simulink model "MBE_Simulation_04_Template_14_11_final"  (R2017b)
settings: Solver=FixedStepAuto  StartTime=0.0  StopTime=inf  FixedStep=0.05  RelTol=1e-3
libraries: simulink x67, canmsglib x4, instrumentlib x2, realtime_pacer_lib x1, hdlsllib x1
(part 4 of 4)

== stateflow chart MBE_Simulation_04_Template_14_11_final/WischerSensorBox/WS_Box_Applikation/WischerSteuerung ==
  state Dummy8 [commented out]
    entry:
    SM_A=true;
    SM_B=false;
    SM_C=false;
    SM_D=false;
    WW_LED=true;
  state Dummy7 [commented out]
    entry:
    SM_A=true;
    SM_B=true;
    SM_C=false;
    SM_D=false;
    WW_LED=true;
  state State_Intervall_Langsam [commented out]
  state State_Wisch_Wasch [commented out]
  state Dummy6 [commented out]
    entry:
    SM_A=true;
    SM_B=false;
    SM_C=false;
    SM_D=true;
    WW_LED=true;
  state Dummy5 [commented out]
    entry:
    SM_A=false;
    SM_B=true;
    SM_C=false;
    SM_D=false;
    WW_LED=true;
  state State_Intervall_Schnell [commented out]
  state State_OFF [commented out]
  state State_Tipp [commented out]
  state Dummy10 [commented out]
    entry:
    SM_A=false;
    SM_B=false;
    SM_C=false;
    SM_D=true;
    WW_LED=true;
  state Dummy11 [commented out]
    entry:
    SM_A=false;
    SM_B=true;
    SM_C=true;
    SM_D=false;
    WW_LED=true;
  state Dummy12 [commented out]
    entry:
    SM_A=false;
    SM_B=false;
    SM_C=true;
    SM_D=true;
    WW_LED=true;
  state Dummy9 [commented out]
    entry:
    SM_A=false;
    SM_B=false;
    SM_C=true;
    SM_D=false;
    WW_LED=true;
  state State_Dauer_Schnell [commented out]
  state State_Dauer_Langsam [commented out]
  state Wischer
    en, du: wisher_cnt = 0
    state Dauer_Schnell
      en, du: wischen = true
      frequency = 0
      wisher_delay = 0
    state Dauer_Langsam
      en, du: wischen = true
      frequency = 0.1
      wisher_delay = 0
    state OFF
      en, du: wischen = false
      wisher_delay = 0
    state Intervall_Langsam
      en, du: wischen = true
      frequency = 0.1
      wisher_delay = 4
    state Intervall_Schnell
      en, du: wischen = true
      frequency = 0.1
      wisher_delay = 2
    state Tipp
      en, du: wischen = true
      frequency = 0
      wisher_delay = 0
    state Wisch_Wasch_Aktivierung
      en, du:
      if SchlossZustand == true
      WischWaschActive = true
      end
      Interrupt = false
      frequency = 0.1
      wisher_delay = 0
      wisher_cnt = 3
    (junction 402) -> Dauer_Schnell [order 3] : [Wischer_Dauer_II]
    (junction 402) -> Dauer_Langsam [order 2] : [Wischer_Dauer_I]
    (junction 402) -> OFF [order 7]
    (default) -> (junction 402)
    Wischer -> (junction 402) [order 1]
    (junction 402) -> Intervall_Langsam [order 5] : [Wischer_Intervall_I]
    (junction 402) -> Intervall_Schnell [order 4] : [Wischer_Intervall_II]
    (junction 402) -> Tipp [order 6] : [Wischer_Tipp]
    (junction 402) -> Wisch_Wasch_Aktivierung [order 1] : [WischWasch || Interrupt]
  state State_MotorWischen1
    en, du: if counter==27
    linkslauf = true
    end
    if WischWasch == true
    Interrupt = true
    end
    state Dummy
      entry:
      SM_A=true;
      SM_B=true;
      SM_C=false;
      SM_D=false;
    state Dummy1
      entry:
      SM_A=false;
      SM_B=true;
      SM_C=true;
      SM_D=false;
    state Dummy3
      entry:
      SM_A=true;
      SM_B=false;
      SM_C=false;
      SM_D=true;
    state Dummy2
      entry:
      SM_A=false;
      SM_B=false;
      SM_C=true;
      SM_D=true;
    (default) -> State_MotorWischen1.Dummy
    State_MotorWischen1.Dummy -> State_MotorWischen1.Dummy1 [order 1] : [linkslauf == 0 && counter <= 27 && after(frequency,sec)]{counter = counter + 1}
    State_MotorWischen1.Dummy1 -> State_MotorWischen1.Dummy [order 2] : [linkslauf == 1 && counter <= 54 && after(frequency,sec)]{counter = counter + 1}
    State_MotorWischen1.Dummy3 -> State_MotorWischen1.Dummy [order 1] : [linkslauf == 0 && counter <= 27 && after(frequency,sec)]{counter = counter + 1}
    State_MotorWischen1.Dummy -> State_MotorWischen1.Dummy3 [order 2] : [linkslauf == 1 && counter <= 54 && after(frequency,sec)]{counter = counter + 1}
    State_MotorWischen1.Dummy2 -> State_MotorWischen1.Dummy1 [order 2] : [linkslauf == 1 && counter <= 54 && after(frequency,sec)]{counter = counter + 1}
    State_MotorWischen1.Dummy1 -> State_MotorWischen1.Dummy2 [order 1] : [linkslauf == 0 && counter <= 27 && after(frequency,sec)]{counter = counter + 1}
    State_MotorWischen1.Dummy3 -> State_MotorWischen1.Dummy2 [order 2] : [linkslauf == 1 && counter <= 54 && after(frequency,sec)]{counter = counter + 1}
    State_MotorWischen1.Dummy2 -> State_MotorWischen1.Dummy3 [order 1] : [linkslauf == 0 && counter <= 27 && after(frequency,sec)]{counter = counter + 1}
  state State_MotorWischen [commented out]
    en, du: WW_LED = true
    if counter==27
    linkslauf = true
    end
    state Dummy [commented out]
      entry:
      SM_A=true;
      SM_B=true;
      SM_C=false;
      SM_D=false;
    state Dummy1 [commented out]
      entry:
      SM_A=false;
      SM_B=true;
      SM_C=true;
      SM_D=false;
    state Dummy3 [commented out]
      entry:
      SM_A=true;
      SM_B=false;
      SM_C=false;
      SM_D=true;
    state Dummy2 [commented out]
      entry:
      SM_A=false;
      SM_B=false;
      SM_C=true;
      SM_D=true;
    (default) -> State_MotorWischen.Dummy [commented out]
    State_MotorWischen.Dummy -> State_MotorWischen.Dummy1 [commented out] : [linkslauf == 0 && counter <= 27 && after(frequency,sec)]{counter = counter + 1}
    State_MotorWischen.Dummy1 -> State_MotorWischen.Dummy [commented out] : [linkslauf == 1 && counter > 0 && after(frequency,sec)]{counter = counter - 1}
    State_MotorWischen.Dummy3 -> State_MotorWischen.Dummy [commented out] : [linkslauf == 0 && counter <= 27 && after(frequency,sec)]{counter = counter + 1}
    State_MotorWischen.Dummy -> State_MotorWischen.Dummy3 [commented out] : [linkslauf == 1 && counter > 0 && after(frequency,sec)]{counter = counter - 1}
    State_MotorWischen.Dummy2 -> State_MotorWischen.Dummy1 [commented out] : [linkslauf == 1 && counter > 0 && after(frequency,sec)]{counter = counter - 1}
    State_MotorWischen.Dummy1 -> State_MotorWischen.Dummy2 [commented out] : [linkslauf == 0 && counter <= 27 && after(frequency,sec)]{counter = counter + 1}
    State_MotorWischen.Dummy3 -> State_MotorWischen.Dummy2 [commented out] : [linkslauf == 1 && counter > 0 && after(frequency,sec)]{counter = counter - 1}
    State_MotorWischen.Dummy2 -> State_MotorWischen.Dummy3 [commented out] : [linkslauf == 0 && counter <= 27 && after(frequency,sec)]{counter = counter + 1}
  state Dummy4 [commented out]
    entry:
    SM_A=true;
    SM_B=false;
    SM_C=true;
    SM_D=false;
    WW_LED=true;
  state State_Delay
  state Wisch_Wasch_LED
    en, du: WW_LED = true
  state Wisch_Wasch
    en, du:
    WW_LED = false
  (default) -> Dummy8 [commented out]
  Dummy6 -> Dummy8 [commented out] : [after(0.5,sec)]
  Dummy8 -> Dummy7 [commented out] : [after(0.5,sec)]
  Dummy7 -> Dummy5 [commented out] : [after(0.5,sec)]
  State_OFF -> State_Wisch_Wasch [commented out]
  State_Wisch_Wasch -> State_OFF [commented out]
  State_OFF -> State_Intervall_Langsam [commented out]
  State_Intervall_Langsam -> State_OFF [commented out]
  Dummy10 -> Dummy6 [commented out] : [after(0.5,sec)]
  (default) -> State_OFF [commented out]
  Dummy5 -> Dummy11 [commented out] : [after(0.5,sec)]
  State_OFF -> State_Intervall_Schnell [commented out]
  State_Intervall_Schnell -> State_OFF [commented out]
  State_Tipp -> State_OFF [commented out]
  State_Dauer_Langsam -> State_OFF [commented out]
  State_OFF -> State_Tipp [commented out] : [Wischer_Tipp == true]
  State_OFF -> State_Dauer_Langsam [commented out]
  State_Dauer_Schnell -> State_OFF [commented out]
  State_OFF -> State_Dauer_Schnell [commented out]
  Dummy12 -> Dummy10 [commented out] : [after(0.5,sec)]
  Dummy11 -> Dummy9 [commented out] : [after(0.5,sec)]
  Dummy9 -> Dummy12 [commented out] : [after(0.5,sec)]
  (default) -> Wischer : {WischWaschActive = false, Interrupt = false}
  (default) -> State_MotorWischen [commented out] : {counter = 0, frequency = 0.1, linkslauf = false}
  Wischer -> State_MotorWischen1 [order 2] : [wischen == true]{counter = 0, linkslauf = false}
  (default) -> Dummy4 [commented out]
  State_MotorWischen1 -> State_Delay : [counter == 55]{wischen = false}
  Wisch_Wasch -> State_MotorWischen1 [order 1] : [wisher_cnt > 0]{counter = 0, linkslauf = false}
  State_Delay -> Wischer [order 2] : after(wisher_delay, sec)
  State_Delay -> Wisch_Wasch [order 1] : [WischWaschActive == true]{wisher_cnt = wisher_cnt - 1}
  Wisch_Wasch -> Wischer [order 2] : [wisher_cnt == 0]{WischWaschActive = false}
  Wischer -> Wisch_Wasch_LED [order 1] : [WischWaschActive == true]
  Wisch_Wasch_LED -> Wisch_Wasch : [after(2,sec)]
  data: Wischer_Tipp input; Wischer_Intervall_I input; Wischer_Intervall_II input; Wischer_Dauer_I input; Wischer_Dauer_II input; WischWasch input; SM_A output; SM_B output; SM_C output; SM_D output; WW_LED output; Steps local; Forward local; StepTime local; StepTime1 local; wisher_delay local double; wisher_cnt local uint8; wisher_dir local boolean; wisher_active local boolean; wisher_timeout local double; frequency local double; counter local double; linkslauf local boolean; Pause local double; wischen local boolean; WischWaschActive local boolean; Interrupt local boolean; SchlossZustand input uint16

== stateflow chart MBE_Simulation_04_Template_14_11_final/WischerSensorBox/WS_Box_Applikation/ScheibenheizungsSteuerung ==
  state State_WaitForDeactivateButton
    entry: SH_LED=false
  state State_OFF
    entry:
    SH_LED=false
  state State_Auto
    entry: SH_LED=true
  state State_Manuell
    entry:
    SH_LED=true
  State_Manuell -> State_WaitForDeactivateButton [order 1] : [after(30,sec)]
  State_WaitForDeactivateButton -> State_OFF : [Scheibenheizung == false]
  (default) -> State_OFF
  State_OFF -> State_Auto [order 2] : [Scheibenheizung_Auto == true && Temperatur < 62]
  State_Manuell -> State_OFF [order 2] : [Scheibenheizung == false]
  State_OFF -> State_Manuell [order 1] : [Scheibenheizung == true]
  State_Auto -> State_OFF : [Scheibenheizung_Auto == false || after(30,sec)]
  data: Scheibenheizung input; Scheibenheizung_Auto input; Temperatur input; SH_LED output

== matlab function MBE_Simulation_04_Template_14_11_final/MLF-VirtualPlatform Setup/Subsystem/Triggered Subsystem/MATLAB Function1 ==
  data: alarmAlarmButton input; alarmAlarmLight input; alarmGenericButton input; alarmGenericLightDown input; alarmGenericLightLeft input; alarmGenericLightRight input; alarmGenericLightUp input; alarmLockButton input; alarmLockLight input; lightBacklight input; lightBrakelight input; lightDaylight input; json_output output size=4096; lightFoglightLeft input; lightFoglightRight input; lightGenericButton input; lightGenericLightDown input; lightGenericLightLeft input; lightGenericLightRight input; lightGenericLightUp input; lightIndicatorLeft input; lightIndicatorRight input; lightLowerBeamHeadlight input; lightReverselight input; lightUpperBeamHeadlight input; windshieldDistanceSensor input; windshieldGenericButton input; windshieldGenericLightDown input; windshieldGenericLightLeft input; windshieldGenericLightRight input; windshieldGenericLightUp input; windshieldHeater input; windshieldLightSensor input; windshieldWasherPump input; windshieldWiperA input; windshieldWiperB input; windshieldWiperC input; windshieldWiperD input
function json_output = fcn( ...
    alarmAlarmButton, ...
    alarmAlarmLight, ...
    alarmGenericButton, ...
    alarmGenericLightDown, ...
    alarmGenericLightLeft, ...
    alarmGenericLightRight, ...
    alarmGenericLightUp, ...
    alarmLockButton, ...
    alarmLockLight, ...
    lightBacklight, ...
    lightBrakelight, ...
    lightDaylight, ...
    lightFoglightLeft, ...
    lightFoglightRight, ...
    lightGenericButton, ...
    lightGenericLightDown, ...
    lightGenericLightLeft, ...
    lightGenericLightRight, ...
    lightGenericLightUp, ...
    lightIndicatorLeft, ...
    lightIndicatorRight, ...
    lightLowerBeamHeadlight, ...
    lightReverselight, ...
    lightUpperBeamHeadlight, ...
    windshieldDistanceSensor, ...
    windshieldGenericButton, ...
    windshieldGenericLightDown, ...
    windshieldGenericLightLeft, ...
    windshieldGenericLightRight, ...
    windshieldGenericLightUp, ...
    windshieldHeater, ...
    windshieldLightSensor, ...
    windshieldWasherPump, ...
    windshieldWiperA, ...
    windshieldWiperB, ...
    windshieldWiperC, ...
    windshieldWiperD)

coder.extrinsic('jsonencode')

% Allocate output array size an initialize with zeroes
json_output = zeros(4096,1,'uint8');


% Prepare the data
json_struct = struct(...
    'alarmAlarmButton', alarmAlarmButton, ...
    'alarmAlarmLight', alarmAlarmLight, ...
    'alarmGenericButton', alarmGenericButton, ...
    'alarmGenericLightDown', alarmGenericLightDown, ...
    'alarmGenericLightLeft', alarmGenericLightLeft, ...
    'alarmGenericLightRight', alarmGenericLightRight, ...
    'alarmGenericLightUp', alarmGenericLightUp, ...
    'alarmLockButton', alarmLockButton, ...
    'alarmLockLight', alarmLockLight, ...
    'lightBacklight',lightBacklight, ...
    'lightBrakelight',lightBrakelight, ...
    'lightDaylight',lightDaylight, ...
    'lightFoglightLeft', lightFoglightLeft, ...
    'lightFoglightRight', lightFoglightRight, ...
    'lightGenericButton', lightGenericButton, ...
    'lightGenericLightDown', lightGenericLightDown, ...
    'lightGenericLightLeft', lightGenericLightLeft, ...
    'lightGenericLightRight', lightGenericLightRight, ...
    'lightGenericLightUp', lightGenericLightUp, ...
    'lightIndicatorLeft', lightIndicatorLeft, ...
    'lightIndicatorRight', lightIndicatorRight, ...
    'lightLowerBeamHeadlight', lightLowerBeamHeadlight, ...
    'lightReverselight', lightReverselight, ...
    'lightUpperBeamHeadlight', lightUpperBeamHeadlight, ...
    'windshieldDistanceSensor', windshieldDistanceSensor, ...
    'windshieldGenericButton', windshieldGenericButton, ...
    'windshieldGenericLightDown', windshieldGenericLightDown, ...
    'windshieldGenericLightLeft', windshieldGenericLightLeft, ...
    'windshieldGenericLightRight', windshieldGenericLightRight, ...
    'windshieldGenericLightUp', windshieldGenericLightUp, ...
    'windshieldHeater', windshieldHeater, ...
    'windshieldLightSensor', windshieldLightSensor, ...
    'windshieldWasherPump', windshieldWasherPump, ...
    'windshieldWiperA', windshieldWiperA, ...
    'windshieldWiperB', windshieldWiperB, ...
    'windshieldWiperC', windshieldWiperC, ...
    'windshieldWiperD', windshieldWiperD ...
)

% Create json string from data
json_string = jsonencode(json_struct)

% Get length of final json string
len = uint16(0)
len = uint16(length(json_string))

% Copy json string char by char to output string
for i = 1:len
    json_output(i) = uint8(json_string(i));
end

json_output(len+1) = uint8(10)

== stateflow chart MBE_Simulation_04_Template_14_11_final/LeuchtenBlinkerBox/LB_Box_Applikation/Steuerung_Licht1 ==
  state on
    state up
      entry:
      up=true;
      left=false;
      right=false;
      down=false;
    state left
      entry:
      up=false;
      left=true;
      right=false;
      down=false;
    state right
      entry:
      up=false;
      left=false;
      right=true;
      down=false;
    state down
      entry:
      up=false;
      left=false;
      right=false;
      down=true;
    (default) -> up
    left -> up : [after(0.5,sec)]
    up -> right : [after(0.5,sec)]
    down -> left : [after(0.5,sec)]
    right -> down : [after(0.5,sec)]
  state off
    entry:
    up=false;
    left=false;
    right=false;
    down=false;
  (default) -> off
  off -> on : [button]
  on -> off : [~button]
  data: down output boolean; left output boolean; right output boolean; up output boolean; button input boolean

== stateflow chart MBE_Simulation_04_Template_14_11_final/SchlossAlarmBox/SA_Box_Applikation/Generic_Lights_Example ==
  state on
    state up
      entry:
      up=true;
      left=false;
      right=false;
      down=false;
    state left
      entry:
      up=false;
      left=true;
      right=false;
      down=false;
    state right
      entry:
      up=false;
      left=false;
      right=true;
      down=false;
    state down
      entry:
      up=false;
      left=false;
      right=false;
      down=true;
    (default) -> up
    left -> up : [after(0.5,sec)]
    up -> right : [after(0.5,sec)]
    down -> left : [after(0.5,sec)]
    right -> down : [after(0.5,sec)]
  state off
    entry:
    up=false;
    left=false;
    right=false;
    down=false;
  (default) -> off
  off -> on : [button]
  on -> off : [~button]
  data: down output boolean; left output boolean; right output boolean; up output boolean; button input boolean

== stateflow chart MBE_Simulation_04_Template_14_11_final/LeuchtenBlinkerBox/LB_Box_Applikation/Generic_Lights_Example ==
  state on
    state up
      entry:
      up=true
      left=false
      right=false
      down=false
    state left
      entry:
      up=false
      left=true
      right=false
      down=false
    state right
      entry:
      up=false
      left=false
      right=true
      down=false
    state down
      entry:
      up=false
      left=false
      right=false
      down=true
    (default) -> up
    left -> up : [after(0.5,sec)]
    up -> right : [after(0.5,sec)]
    down -> left : [after(0.5,sec)]
    right -> down : [after(0.5,sec)]
  state off
    entry:
    up=false
    left=false
    right=false
    down=false
  (default) -> off
  off -> on : [button]
  on -> off : [~button]
  data: down output boolean; left output boolean; right output boolean; up output boolean; button input boolean

== stateflow chart MBE_Simulation_04_Template_14_11_final/WischerSensorBox/WS_Box_Applikation/Generic_Lights_Example ==
  state on
    state up
      entry:
      up=true;
      left=false;
      right=false;
      down=false;
    state left
      entry:
      up=false;
      left=true;
      right=false;
      down=false;
    state right
      entry:
      up=false;
      left=false;
      right=true;
      down=false;
    state down
      entry:
      up=false;
      left=false;
      right=false;
      down=true;
    (default) -> up
    left -> up : [after(0.5,sec)]
    up -> right : [after(0.5,sec)]
    down -> left : [after(0.5,sec)]
    right -> down : [after(0.5,sec)]
  state off
    entry:
    up=false;
    left=false;
    right=false;
    down=false;
  (default) -> off
  off -> on : [button]
  on -> off : [~button]
  data: down output boolean; left output boolean; right output boolean; up output boolean; button input boolean

== matlab function MBE_Simulation_04_Template_14_11_final/MLF-VirtualPlatform Setup/Subsystem2/Triggered Subsystem/MATLAB Function ==
  data: json_input input; alarmAlarmButton output; alarmAlarmLight output; alarmGenericButton output; alarmGenericLightDown output; alarmGenericLightLeft output; alarmGenericLightRight output; alarmGenericLightUp output; alarmLockButton output; alarmLockLight output; cockpitAlarmReset output; cockpitBrake output; cockpitIgnition output; cockpitIndicator output; cockpitLightSwitch output; cockpitSteeringAngleDeg output; cockpitTemperature output; cockpitVelocity output; cockpitWarnLight output; cockpitWindshieldHeater output; cockpitWindshieldWasherMode output; cockpitWindshieldWasherPump output; lightBacklight output; lightBrakelight output; lightDaylight output; lightFoglightLeft output; lightFoglightRight output; lightGenericButton output; lightGenericLightDown output; lightGenericLightLeft output; lightGenericLightRight output; lightGenericLightUp output; lightIndicatorLeft output; lightIndicatorRight output; lightLowerBeamHeadlight output; lightReverselight output; lightUpperBeamHeadlight output; windshieldDistanceSensor output; windshieldGenericButton output; windshieldGenericLightDown output; windshieldGenericLightLeft output; windshieldGenericLightRight output; windshieldGenericLightUp output; windshieldHeater output; windshieldLightSensor output; windshieldWasherPump output; windshieldWiperA output; windshieldWiperB output; windshieldWiperC output; windshieldWiperD output
function [ ...
    alarmAlarmButton, ...
    alarmAlarmLight, ...
    alarmGenericButton, ...
    alarmGenericLightDown, ...
    alarmGenericLightLeft, ...
    alarmGenericLightRight, ...
    alarmGenericLightUp, ...
    alarmLockButton, ...
    alarmLockLight, ...
    cockpitAlarmReset, ...
    cockpitBrake, ...
    cockpitIgnition, ...
    cockpitIndicator, ...
    cockpitLightSwitch, ...
    cockpitSteeringAngleDeg, ...
    cockpitTemperature, ...
    cockpitVelocity, ...
    cockpitWarnLight, ...
    cockpitWindshieldHeater, ...
    cockpitWindshieldWasherMode, ...
    cockpitWindshieldWasherPump, ...
    lightBacklight, ...
    lightBrakelight, ...
    lightDaylight, ...
    lightFoglightLeft, ...
    lightFoglightRight, ...
    lightGenericButton, ...
    lightGenericLightDown, ...
    lightGenericLightLeft, ...
    lightGenericLightRight, ...
    lightGenericLightUp, ...
    lightIndicatorLeft, ...
    lightIndicatorRight, ...
    lightLowerBeamHeadlight, ...
    lightReverselight, ...
    lightUpperBeamHeadlight, ...
    windshieldDistanceSensor, ...
    windshieldGenericButton, ...
    windshieldGenericLightDown, ...
    windshieldGenericLightLeft, ...
    windshieldGenericLightRight, ...
    windshieldGenericLightUp, ...
    windshieldHeater, ...
    windshieldLightSensor, ...
    windshieldWasherPump, ...
    windshieldWiperA, ...
    windshieldWiperB, ...
    windshieldWiperC, ...
    windshieldWiperD ...
    ] = fcn(json_input)

coder.extrinsic('jsondecode');

%bar = '{"alarmAlarmButton": false,"lightBacklight": true,"lightBrakelight": true,"lightDaylight": true}    '

jsonLen = 0;

for i = 1:length(json_input)
   c = json_input(i);
   if c == 0
        break;
   else
        jsonLen = i;
   end
   
end

chr = blanks(jsonLen);

for i = 1:jsonLen
    chr(i) = json_input(i);
end

jsonStruct.alarmAlarmButton = false;
jsonStruct.alarmAlarmLight = false;
jsonStruct.alarmGenericButton = false;
jsonStruct.alarmGenericLightDown = false;
jsonStruct.alarmGenericLightLeft = false;
jsonStruct.alarmGenericLightRight = false;
jsonStruct.alarmGenericLightUp = false;
jsonStruct.alarmLockButton = false;
jsonStruct.alarmLockLight = false;
jsonStruct.cockpitAlarmReset = double(0);
jsonStruct.cockpitBrake = double(0);
jsonStruct.cockpitIgnition = double(0);
jsonStruct.cockpitIndicator = double(0);
jsonStruct.cockpitLightSwitch = double(0);
jsonStruct.cockpitSteeringAngleDeg = double(0);
jsonStruct.cockpitTemperature = double(0);
jsonStruct.cockpitVelocity = double(0);
jsonStruct.cockpitWarnLight = double(0);
jsonStruct.cockpitWindshieldHeater = double(0);
jsonStruct.cockpitWindshieldWasherMode = double(0);
jsonStruct.cockpitWindshieldWasherPump = double(0);
jsonStruct.lightBacklight = false;
jsonStruct.lightBrakelight = false;
jsonStruct.lightDaylight = false;
jsonStruct.lightFoglightLeft = false;
jsonStruct.lightFoglightRight = false;
jsonStruct.lightGenericButton = false;
jsonStruct.lightGenericLightDown = false;
jsonStruct.lightGenericLightLeft = false;
jsonStruct.lightGenericLightRight = false;
jsonStruct.lightGenericLightUp = false;
jsonStruct.lightIndicatorLeft = false;
jsonStruct.lightIndicatorRight = false;
jsonStruct.lightLowerBeamHeadlight = false;
jsonStruct.lightReverselight = false;
jsonStruct.lightUpperBeamHeadlight = false;
jsonStruct.windshieldDistanceSensor = double(0);
jsonStruct.windshieldGenericButton = false;
jsonStruct.windshieldGenericLightDown = false;
jsonStruct.windshieldGenericLightLeft = false;
jsonStruct.windshieldGenericLightRight = false;
jsonStruct.windshieldGenericLightUp = false;
jsonStruct.windshieldHeater = false;
jsonStruct.windshieldLightSensor = false;
jsonStruct.windshieldWasherPump = false;
jsonStruct.windshieldWiperA = false;
jsonStruct.windshieldWiperB = false;
jsonStruct.windshieldWiperC = false;
jsonStruct.windshieldWiperD = false;

jsonStruct = jsondecode(chr);

alarmAlarmButton = jsonStruct.alarmAlarmButton;
alarmAlarmLight = jsonStruct.alarmAlarmLight;
alarmGenericButton = jsonStruct.alarmGenericButton;
alarmGenericLightDown = jsonStruct.alarmGenericLightDown;
alarmGenericLightLeft = jsonStruct.alarmGenericLightLeft;
alarmGenericLightRight = jsonStruct.alarmGenericLightRight;
alarmGenericLightUp = jsonStruct.alarmGenericLightUp;
alarmLockButton = jsonStruct.alarmLockButton;
alarmLockLight = jsonStruct.alarmLockLight;
cockpitAlarmReset = jsonStruct.cockpitAlarmReset;
cockpitBrake = jsonStruct.cockpitBrake;
cockpitIgnition = jsonStruct.cockpitIgnition;
cockpitIndicator = jsonStruct.cockpitIndicator;
cockpitLightSwitch = jsonStruct.cockpitLightSwitch;
cockpitSteeringAngleDeg = jsonStruct.cockpitSteeringAngleDeg;
cockpitTemperature = jsonStruct.cockpitTemperature;
cockpitVelocity = jsonStruct.cockpitVelocity;
cockpitWarnLight = jsonStruct.cockpitWarnLight;
cockpitWindshieldHeater = jsonStruct.cockpitWindshieldHeater;
cockpitWindshieldWasherMode = jsonStruct.cockpitWindshieldWasherMode;
cockpitWindshieldWasherPump = jsonStruct.cockpitWindshieldWasherPump;
lightBacklight = jsonStruct.lightBacklight;
lightBrakelight = jsonStruct.lightBrakelight;
lightDaylight = jsonStruct.lightDaylight;
lightFoglightLeft = jsonStruct.lightFoglightLeft;
lightFoglightRight = jsonStruct.lightFoglightRight;
lightGenericButton = jsonStruct.lightGenericButton;
lightGenericLightDown = jsonStruct.lightGenericLightDown;
lightGenericLightLeft = jsonStruct.lightGenericLightLeft;
lightGenericLightRight = jsonStruct.lightGenericLightRight;
lightGenericLightUp = jsonStruct.lightGenericLightUp;
lightIndicatorLeft = jsonStruct.lightIndicatorLeft;
lightIndicatorRight = jsonStruct.lightIndicatorRight;
lightLowerBeamHeadlight = jsonStruct.lightLowerBeamHeadlight;
lightReverselight = jsonStruct.lightReverselight;
lightUpperBeamHeadlight = jsonStruct.lightUpperBeamHeadlight;
windshieldDistanceSensor = jsonStruct.windshieldDistanceSensor;
windshieldGenericButton = jsonStruct.windshieldGenericButton;
windshieldGenericLightDown = jsonStruct.windshieldGenericLightDown;
windshieldGenericLightLeft = jsonStruct.windshieldGenericLightLeft;
windshieldGenericLightRight = jsonStruct.windshieldGenericLightRight;
windshieldGenericLightUp = jsonStruct.windshieldGenericLightUp;
windshieldHeater = jsonStruct.windshieldHeater;
windshieldLightSensor = jsonStruct.windshieldLightSensor;
windshieldWasherPump = jsonStruct.windshieldWasherPump;
windshieldWiperA = jsonStruct.windshieldWiperA;
windshieldWiperB = jsonStruct.windshieldWiperB;
windshieldWiperC = jsonStruct.windshieldWiperC;
windshieldWiperD = jsonStruct.windshieldWiperD;
